simulink model "Esm"  (R2025b)
settings: Solver=FixedStepDiscrete  StartTime=0.0  StopTime=0.010  FixedStep=0.001  RelTol=1e-3
settings Model: Creator=leeyj  LastModifiedBy=leeyj

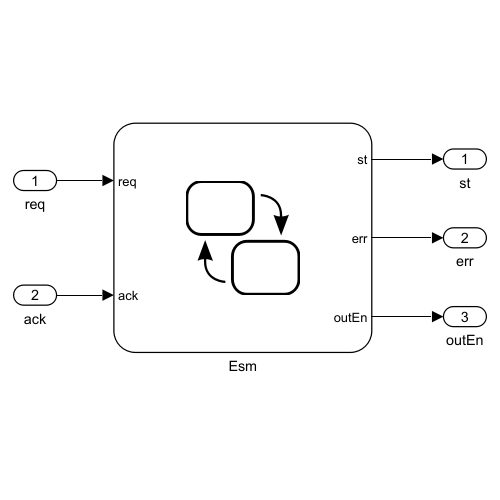
[thumbnail: Simulink's stored preview of the top-level diagram]
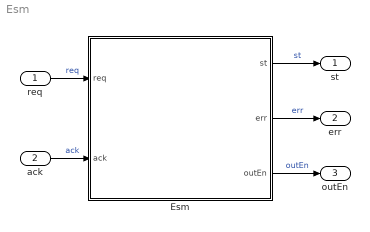
== system Esm ==
  req : Inport  OutDataTypeStr=uint8  Interpolate=off
  ack : Inport  Port=2  OutDataTypeStr=boolean  Interpolate=off
  Esm : Stateflow chart  TreatAsAtomicUnit=on
  st : Outport
  err : Outport  Port=2
  outEn : Outport  Port=3
  wires:
  ack/1 -> Esm/2(ack)  "ack"
  req/1 -> Esm/1(req)  "req"
  Esm/1(st) -> st/1  "st"
  Esm/3(outEn) -> outEn/1  "outEn"
  Esm/2(err) -> err/1  "err"

== stateflow chart Esm/Esm ==
  settings: updateMethod=DISCRETE  sampleTime=0.001
  state Al
    during:
    err = err && !ack;
    state Init
      entry: st = 1;
      during:
      err = err || (req != 0 && req != 1);
    state PreOp
      entry: st = 2;
      during:
      err = err || (req != 0 && req != 2);
    state SafeOp
      entry: st = 4;
      during:
      err = err || (req != 0 && req != 4);
    state Op
      entry: st = 8; outEn = true;
      during:
      err = err || (req != 0 && req != 8);
      exit: outEn = false;
    (default) -> Init
    SafeOp -> Init [order 1] : [req == 1]
    Op -> Init [order 1] : [req == 1]
    Init -> PreOp : [req == 2 && !err]
    PreOp -> Init [order 1] : [req == 1]
    Op -> PreOp [order 2] : [req == 2 && !err]
    PreOp -> SafeOp [order 2] : [req == 4 && !err]
    SafeOp -> PreOp [order 2] : [req == 2 && !err]
    SafeOp -> Op [order 3] : [req == 8 && !err]
    Op -> SafeOp [order 3] : [req == 4 && !err]
  (default) -> Al
  data: req input uint8; ack input boolean; st output uint8; err output boolean; outEn output boolean
